simulink model "Lorien"  (R2014a)
settings: Solver=ode45  StartTime=0.0  StopTime=inf  FixedStep=0.05  RelTol=1e-3
undefined symbols (not defined in the file or in its folder): dotSelection
settings Model: Creator=Ilya  LastModifiedBy=Ilya
settings OptimizationCC: InitFltsAndDblsToZero=on
settings DebuggingCC: SaveWithParameterizedLinksMsg=none  UnderspecifiedInitializationDetection=Classic  SignalResolutionControl=TryResolveAllWithWarning  MultiTaskDSMMsg=warning  MultiTaskCondExecSysMsg=none
settings SFSimCC: SimParseCustomCode=off
settings RTWCC: IncludeERTFirstTime=on
settings GRTTargetCC: TargetFcnLib=ansi_tfl_tmw.mat  CombineOutputUpdateFcns=off  GRTInterface=on

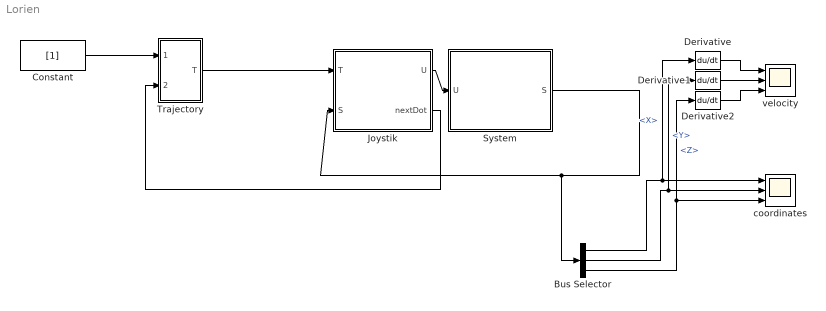
== system Lorien ==
  Bus Selector : BusSelector  DialogController=Simulink.DDGSource_Bus  OutputSignals=X,Y,Z
  Constant : Constant  Value=[1]
  Derivative : Derivative
  Derivative1 : Derivative
  Derivative2 : Derivative
  "Joystik " : Subsystem
  System : Subsystem  mask{X0=[10, 25, 2], WorkArea=[50, 20, 15], Platform=[2, 1.2]}
      mask prompts: X0 "Initial position [x, y, z] (m)"; WorkArea "Work area size [a, b, h] (m)"; Platform "Platform size [d, f]"
      mask init:
      | a = WorkArea(1);
      | b = WorkArea(2);
      | h = WorkArea(3);
      | 
      | d = Platform(1);
      | f = Platform(2);
      | 
      | L0 = iSolver(X0, a, b, d, f, h);
  Trajectory : Subsystem  mask{i=1}
      mask prompts: i "Iteration [i]"
  coordinates : Scope  NumInputPorts=3
      settings: TimeRange=10  YMin=9.5~23.75~0.967081  YMax=10.5~26.25~1.06888  SaveName=ScopeData2
  velocity : Scope  NumInputPorts=3
      settings: TimeRange=10  YMin=9.75~-5~4.975  YMax=11.75~5~5.2
  wires:
  "Joystik "/1(U) -> System/1(U)
  System/1(S) -> "Joystik "/2(S), Bus Selector/1
  Bus Selector/1 -> Derivative/1, coordinates/1  "<X>"
  Bus Selector/2 -> Derivative1/1, coordinates/2  "<Y>"
  Bus Selector/3 -> coordinates/3, Derivative2/1  "<Z>"
  Derivative/1 -> velocity/1
  Derivative1/1 -> velocity/2
  Derivative2/1 -> velocity/3
  Constant/1 -> Trajectory/1(trSelect)
  "Joystik "/2(nextDot) -> Trajectory/2(nextDot)
  Trajectory/1(T) -> "Joystik "/1(T)

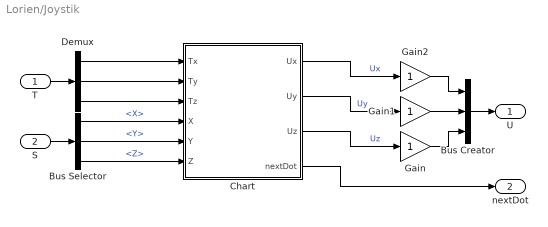
== system Lorien/Joystik  ==
  T : Inport
  S : Inport  Port=2
  Bus Creator : BusCreator  DialogController=Simulink.DDGSource_Bus  Inputs=3
  Bus Selector : BusSelector  DialogController=Simulink.DDGSource_Bus  OutputSignals=X,Y,Z
  Chart : Stateflow chart  TreatAsAtomicUnit=on
  Demux : Demux  Outputs=3
  Gain : Gain
  Gain1 : Gain
  Gain2 : Gain
  U : Outport
  nextDot : Outport  Port=2
  wires:
  Bus Creator/1 -> U/1
  S/1 -> Bus Selector/1
  Bus Selector/1 -> Chart/4(X)  "<X>"
  Bus Selector/2 -> Chart/5(Y)  "<Y>"
  Bus Selector/3 -> Chart/6(Z)  "<Z>"
  Chart/1(Ux) -> Gain2/1  "Ux"
  Chart/2(Uy) -> Gain1/1  "Uy"
  Chart/3(Uz) -> Gain/1  "Uz"
  T/1 -> Demux/1
  Demux/1 -> Chart/1(Tx)
  Demux/2 -> Chart/2(Ty)
  Demux/3 -> Chart/3(Tz)
  Gain/1 -> Bus Creator/3
  Gain1/1 -> Bus Creator/2
  Gain2/1 -> Bus Creator/1
  Chart/4(nextDot) -> nextDot/1

== system Lorien/System ==
  U : Inport
  Controller : Subsystem
  Kranes : Subsystem
      mask init:
      | T=0.1;
  Monitor : Subsystem  mask{B=on, X0=X0, A=WorkArea, P=Platform, S=15, U=1}
      mask prompts: B "Enable animation"; X0 "Initial position [x,y,z] (m)"; A "Area size [a, b, h] (m)"; P "Platform size [f, d] (m)"; S "Scale"; U "Update time (sec)"
      mask init:
      | Config.a = A(1);
      | Config.b = A(2);
      | Config.h = A(3);
      | Config.f = P(1);
      | Config.d = P(2);
      | Config.E = B;
      | Config.S = S;
      | Config.U = U;
      | Config.X0 = X0;
  S : Outport
  wires:
  Controller/1(Q) -> Kranes/1(Q)
  Kranes/1(L) -> Controller/1(L)
  Controller/2(S) -> S/1, Monitor/1(S)
  U/1 -> Controller/2(U)

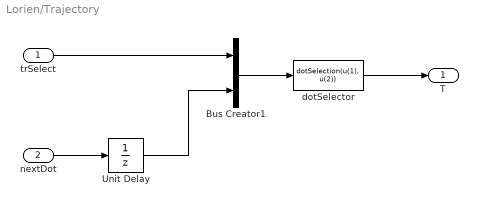
== system Lorien/Trajectory ==
  trSelect : Inport
  nextDot : Inport  Port=2
  Bus Creator1 : BusCreator  Inputs=2
  Unit Delay : UnitDelay  SampleTime=-1
  dotSelector : MATLABFcn  MATLABFcn=dotSelection(u(1), u(2))  OutputDimensions=3
  T : Outport
  wires:
  nextDot/1 -> Unit Delay/1
  Unit Delay/1 -> Bus Creator1/2
  trSelect/1 -> Bus Creator1/1
  dotSelector/1 -> T/1
  Bus Creator1/1 -> dotSelector/1

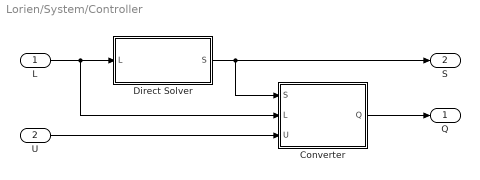
== system Lorien/System/Controller ==
  L : Inport
  U : Inport  Port=2
  Converter : Subsystem
  Direct Solver : Subsystem
  Q : Outport
  S : Outport  Port=2
  wires:
  U/1 -> Converter/3(U)
  Converter/1(Q) -> Q/1
  L/1 -> Direct Solver/1(L), Converter/2(L)
  Direct Solver/1(S) -> S/1, Converter/1(S)

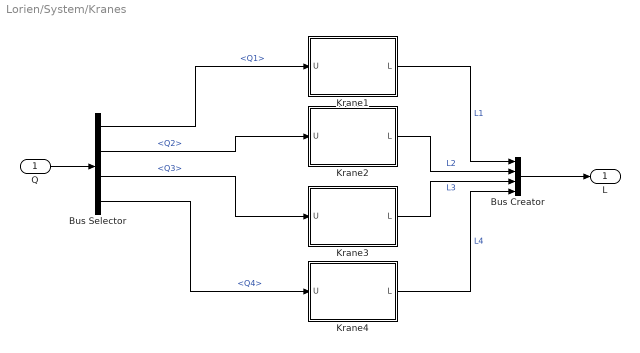
== system Lorien/System/Kranes ==
  Q : Inport
  Bus Creator : BusCreator  DialogController=Simulink.DDGSource_Bus
  Bus Selector : BusSelector  DialogController=Simulink.DDGSource_Bus  OutputSignals=Q1,Q2,Q3,Q4
  Krane1 : Subsystem  mask{IC=L0(1), T=T, D=0.5}
      mask prompts: IC "Initial condition"; D "Winch diameter (m)"
  Krane2 : Subsystem  mask{IC=L0(1), T=T, D=0.5}
      mask prompts: IC "Initial condition"; D "Winch diameter (m)"
  Krane3 : Subsystem  mask{IC=L0(1), T=T, D=0.5}
      mask prompts: IC "Initial condition"; D "Winch diameter (m)"
  Krane4 : Subsystem  mask{IC=L0(1), T=T, D=0.5}
      mask prompts: IC "Initial condition"; D "Winch diameter (m)"
  L : Outport
  wires:
  Bus Creator/1 -> L/1
  Krane1/1(L) -> Bus Creator/1  "L1"
  Krane2/1(L) -> Bus Creator/2  "L2"
  Krane3/1(L) -> Bus Creator/3  "L3"
  Krane4/1(L) -> Bus Creator/4  "L4"
  Q/1 -> Bus Selector/1
  Bus Selector/1 -> Krane1/1(U)  "<Q1>"
  Bus Selector/2 -> Krane2/1(U)  "<Q2>"
  Bus Selector/3 -> Krane3/1(U)  "<Q3>"
  Bus Selector/4 -> Krane4/1(U)  "<Q4>"

== system Lorien/System/Monitor ==
  S : Inport
  S-Function : S-Function  FunctionName=Animation  Parameters=Config  EnableBusSupport=off
  wires:
  S/1 -> S-Function/1

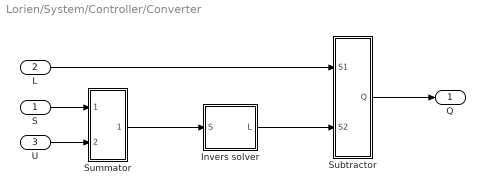
== system Lorien/System/Controller/Converter ==
  S : Inport
  L : Inport  Port=2
  U : Inport  Port=3
  Invers solver : Subsystem
  Subtractor : Subsystem
      mask Display: disp('sub')
  Summator : Subsystem
      mask Display: disp('sum')
  Q : Outport
  wires:
  Summator/1(SUM) -> Invers solver/1(S)
  Invers solver/1(L) -> Subtractor/2(S2)
  S/1 -> Summator/1(S1)
  L/1 -> Subtractor/1(S1)
  Subtractor/1(Q) -> Q/1
  U/1 -> Summator/2(S2)

== system Lorien/System/Controller/Direct Solver ==
  L : Inport
  Bus Creator : BusCreator  DialogController=Simulink.DDGSource_Bus  Inputs=3
  Demux : Demux  Outputs=3
  MATLAB Fcn : MATLABFcn  MATLABFcn=dSolver(u, a, b, d, f, h)  OutputDimensions=3
  S : Outport
  wires:
  L/1 -> MATLAB Fcn/1
  MATLAB Fcn/1 -> Demux/1
  Demux/1 -> Bus Creator/1  "X"
  Demux/2 -> Bus Creator/2  "Y"
  Demux/3 -> Bus Creator/3  "Z"
  Bus Creator/1 -> S/1

== system Lorien/System/Kranes/Krane1 ==
  U : Inport
  Motor : Subsystem
      mask Display: plot(-80,-80,80,80,[0,9,18,24,29,30,29,24,18,9,0,-9,-18,-24,-29,-30,-29,-24,-18,-9,0],[30,29,24,18,9,0,-9,-18,-24,-29,-30,-29,-24,-18,-9,0,9,18,24,29,30],[-29,-35,-35,-29],[-8,-8,8,8],[29,35,35,29],[-8,-8,8,8],[-35,-55],[0,0],[35,55],[0,0],[-78,-50,-50,-49,-45,-39,-33,-26,-21,-18,-17,-19,-22,-22,-26,-27,-25,-22,-16,-9,-3,2,6,6,4,1,1,-3,-4,-2,2,7,14,20,26,29,30,28,24,24,21,20,21,25,31,37,44,49,50,50,50,78]*.7,[58,58,57.2,49.2,42.8,38.8,38,39.6,44.4,51.6,59.6,67.6,72.4,72.4,65.2,57.2,49.2,42.8,38.8,38,39.6,44.4,51.6,59.6,67.6,72.4,72.4,65.2,57.2,49.2,42.8,38.8,38,39.6,44.4,51.6,59.6,67.6,72.4,72.4,65.2,57.2,49.2,42.8,38.8,38,39.6,44.4,51.6,58,58,58]*.6+15 );
  Winch : Subsystem
  L : Outport
  wires:
  Motor/1(Alpha) -> Winch/1(Alpha)
  Winch/1(L) -> L/1
  U/1 -> Motor/1(U)

== system Lorien/System/Kranes/Krane2 ==
  U : Inport
  Motor : Subsystem
      mask Display: plot(-80,-80,80,80,[0,9,18,24,29,30,29,24,18,9,0,-9,-18,-24,-29,-30,-29,-24,-18,-9,0],[30,29,24,18,9,0,-9,-18,-24,-29,-30,-29,-24,-18,-9,0,9,18,24,29,30],[-29,-35,-35,-29],[-8,-8,8,8],[29,35,35,29],[-8,-8,8,8],[-35,-55],[0,0],[35,55],[0,0],[-78,-50,-50,-49,-45,-39,-33,-26,-21,-18,-17,-19,-22,-22,-26,-27,-25,-22,-16,-9,-3,2,6,6,4,1,1,-3,-4,-2,2,7,14,20,26,29,30,28,24,24,21,20,21,25,31,37,44,49,50,50,50,78]*.7,[58,58,57.2,49.2,42.8,38.8,38,39.6,44.4,51.6,59.6,67.6,72.4,72.4,65.2,57.2,49.2,42.8,38.8,38,39.6,44.4,51.6,59.6,67.6,72.4,72.4,65.2,57.2,49.2,42.8,38.8,38,39.6,44.4,51.6,59.6,67.6,72.4,72.4,65.2,57.2,49.2,42.8,38.8,38,39.6,44.4,51.6,58,58,58]*.6+15 );
  Winch : Subsystem
  L : Outport
  wires:
  U/1 -> Motor/1(U)
  Winch/1(L) -> L/1
  Motor/1(Alpha) -> Winch/1(Alpha)

== system Lorien/System/Kranes/Krane3 ==
  U : Inport
  Motor : Subsystem
      mask Display: plot(-80,-80,80,80,[0,9,18,24,29,30,29,24,18,9,0,-9,-18,-24,-29,-30,-29,-24,-18,-9,0],[30,29,24,18,9,0,-9,-18,-24,-29,-30,-29,-24,-18,-9,0,9,18,24,29,30],[-29,-35,-35,-29],[-8,-8,8,8],[29,35,35,29],[-8,-8,8,8],[-35,-55],[0,0],[35,55],[0,0],[-78,-50,-50,-49,-45,-39,-33,-26,-21,-18,-17,-19,-22,-22,-26,-27,-25,-22,-16,-9,-3,2,6,6,4,1,1,-3,-4,-2,2,7,14,20,26,29,30,28,24,24,21,20,21,25,31,37,44,49,50,50,50,78]*.7,[58,58,57.2,49.2,42.8,38.8,38,39.6,44.4,51.6,59.6,67.6,72.4,72.4,65.2,57.2,49.2,42.8,38.8,38,39.6,44.4,51.6,59.6,67.6,72.4,72.4,65.2,57.2,49.2,42.8,38.8,38,39.6,44.4,51.6,59.6,67.6,72.4,72.4,65.2,57.2,49.2,42.8,38.8,38,39.6,44.4,51.6,58,58,58]*.6+15 );
  Winch : Subsystem
  L : Outport
  wires:
  Motor/1(Alpha) -> Winch/1(Alpha)
  Winch/1(L) -> L/1
  U/1 -> Motor/1(U)

== system Lorien/System/Kranes/Krane4 ==
  U : Inport
  Motor : Subsystem
      mask Display: plot(-80,-80,80,80,[0,9,18,24,29,30,29,24,18,9,0,-9,-18,-24,-29,-30,-29,-24,-18,-9,0],[30,29,24,18,9,0,-9,-18,-24,-29,-30,-29,-24,-18,-9,0,9,18,24,29,30],[-29,-35,-35,-29],[-8,-8,8,8],[29,35,35,29],[-8,-8,8,8],[-35,-55],[0,0],[35,55],[0,0],[-78,-50,-50,-49,-45,-39,-33,-26,-21,-18,-17,-19,-22,-22,-26,-27,-25,-22,-16,-9,-3,2,6,6,4,1,1,-3,-4,-2,2,7,14,20,26,29,30,28,24,24,21,20,21,25,31,37,44,49,50,50,50,78]*.7,[58,58,57.2,49.2,42.8,38.8,38,39.6,44.4,51.6,59.6,67.6,72.4,72.4,65.2,57.2,49.2,42.8,38.8,38,39.6,44.4,51.6,59.6,67.6,72.4,72.4,65.2,57.2,49.2,42.8,38.8,38,39.6,44.4,51.6,59.6,67.6,72.4,72.4,65.2,57.2,49.2,42.8,38.8,38,39.6,44.4,51.6,58,58,58]*.6+15 );
  Winch : Subsystem
  L : Outport
  wires:
  U/1 -> Motor/1(U)
  Winch/1(L) -> L/1
  Motor/1(Alpha) -> Winch/1(Alpha)

== system Lorien/System/Controller/Converter/Invers solver ==
  S : Inport
  Bus Creator : BusCreator  DialogController=Simulink.DDGSource_Bus
  Demux : Demux
  MATLAB Fcn : MATLABFcn  MATLABFcn=iSolver(u, a, b, d, f, h)  OutputDimensions=4
  L : Outport
  wires:
  Demux/1 -> Bus Creator/1  "L1"
  Demux/2 -> Bus Creator/2  "L2"
  Demux/3 -> Bus Creator/3  "L3"
  Demux/4 -> Bus Creator/4  "L4"
  Bus Creator/1 -> L/1
  S/1 -> MATLAB Fcn/1
  MATLAB Fcn/1 -> Demux/1

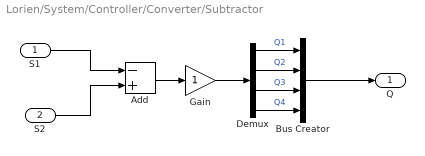
== system Lorien/System/Controller/Converter/Subtractor ==
  S1 : Inport
  S2 : Inport  Port=2
  Add : Sum  Inputs=-+
  Bus Creator : BusCreator  DialogController=Simulink.DDGSource_Bus
  Demux : Demux
  Gain : Gain
  Q : Outport
  wires:
  Demux/3 -> Bus Creator/3  "Q3"
  Demux/2 -> Bus Creator/2  "Q2"
  Demux/1 -> Bus Creator/1  "Q1"
  Add/1 -> Gain/1
  S2/1 -> Add/2
  S1/1 -> Add/1
  Demux/4 -> Bus Creator/4  "Q4"
  Gain/1 -> Demux/1
  Bus Creator/1 -> Q/1

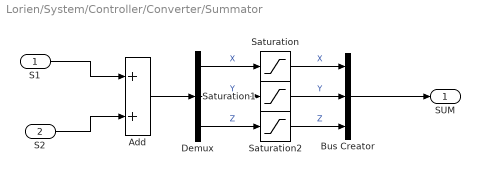
== system Lorien/System/Controller/Converter/Summator ==
  S1 : Inport
  S2 : Inport  Port=2
  Add : Sum
  Bus Creator : BusCreator  DialogController=Simulink.DDGSource_Bus  Inputs=3
  Demux : Demux  Outputs=3
  Saturation : Saturate  UpperLimit=b-f/2  LowerLimit=f/2
  Saturation1 : Saturate  UpperLimit=a-d/2  LowerLimit=d/2
  Saturation2 : Saturate  UpperLimit=h  LowerLimit=0
  SUM : Outport
  wires:
  S1/1 -> Add/1
  S2/1 -> Add/2
  Add/1 -> Demux/1
  Bus Creator/1 -> SUM/1
  Demux/1 -> Saturation/1  "X"
  Demux/2 -> Saturation1/1  "Y"
  Demux/3 -> Saturation2/1  "Z"
  Saturation/1 -> Bus Creator/1  "X"
  Saturation1/1 -> Bus Creator/2  "Y"
  Saturation2/1 -> Bus Creator/3  "Z"

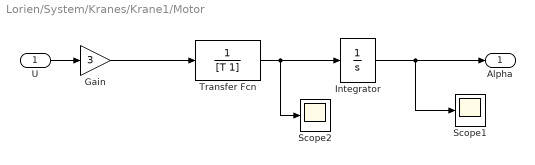
== system Lorien/System/Kranes/Krane1/Motor ==
  U : Inport
  Gain : Gain  Gain=3
  Integrator : Integrator  InitialCondition=2*IC/D
  Scope1 : Scope
      settings: YMin=111.659  YMax=111.659
  Scope2 : Scope
      settings: YMin=2.47e-010  YMax=2.555e-010  SaveName=ScopeData3
  Transfer Fcn : TransferFcn  Denominator=[T 1]
  Alpha : Outport
  wires:
  U/1 -> Gain/1
  Integrator/1 -> Alpha/1, Scope1/1
  Gain/1 -> Transfer Fcn/1
  Transfer Fcn/1 -> Integrator/1, Scope2/1

== system Lorien/System/Kranes/Krane1/Winch ==
  Alpha : Inport
  Gain : Gain  Gain=D/2
  L : Outport
  wires:
  Alpha/1 -> Gain/1
  Gain/1 -> L/1

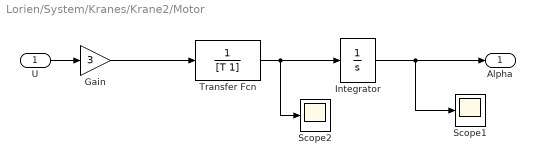
== system Lorien/System/Kranes/Krane2/Motor ==
  U : Inport
  Gain : Gain  Gain=3
  Integrator : Integrator  InitialCondition=2*IC/D
  Scope1 : Scope
  Scope2 : Scope
      settings: YMin=2.47e-010  YMax=2.555e-010  SaveName=ScopeData3
  Transfer Fcn : TransferFcn  Denominator=[T 1]
  Alpha : Outport
  wires:
  Transfer Fcn/1 -> Scope2/1, Integrator/1
  Gain/1 -> Transfer Fcn/1
  Integrator/1 -> Scope1/1, Alpha/1
  U/1 -> Gain/1

== system Lorien/System/Kranes/Krane2/Winch ==
  Alpha : Inport
  Gain : Gain  Gain=D/2
  L : Outport
  wires:
  Gain/1 -> L/1
  Alpha/1 -> Gain/1

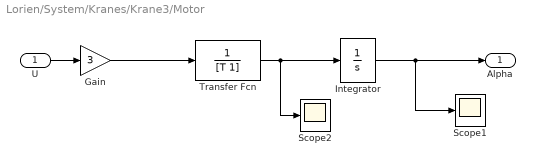
== system Lorien/System/Kranes/Krane3/Motor ==
  U : Inport
  Gain : Gain  Gain=3
  Integrator : Integrator  InitialCondition=2*IC/D
  Scope1 : Scope
  Scope2 : Scope
      settings: YMin=2.47e-010  YMax=2.555e-010  SaveName=ScopeData3
  Transfer Fcn : TransferFcn  Denominator=[T 1]
  Alpha : Outport
  wires:
  U/1 -> Gain/1
  Integrator/1 -> Alpha/1, Scope1/1
  Gain/1 -> Transfer Fcn/1
  Transfer Fcn/1 -> Integrator/1, Scope2/1

== system Lorien/System/Kranes/Krane3/Winch ==
  Alpha : Inport
  Gain : Gain  Gain=D/2
  L : Outport
  wires:
  Alpha/1 -> Gain/1
  Gain/1 -> L/1

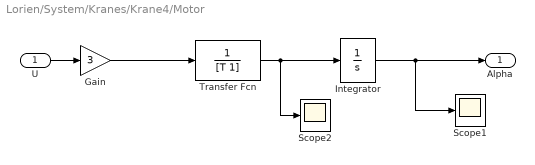
== system Lorien/System/Kranes/Krane4/Motor ==
  U : Inport
  Gain : Gain  Gain=3
  Integrator : Integrator  InitialCondition=2*IC/D
  Scope1 : Scope
  Scope2 : Scope
      settings: YMin=2.47e-010  YMax=2.555e-010  SaveName=ScopeData3
  Transfer Fcn : TransferFcn  Denominator=[T 1]
  Alpha : Outport
  wires:
  Transfer Fcn/1 -> Scope2/1, Integrator/1
  Gain/1 -> Transfer Fcn/1
  Integrator/1 -> Scope1/1, Alpha/1
  U/1 -> Gain/1

== system Lorien/System/Kranes/Krane4/Winch ==
  Alpha : Inport
  Gain : Gain  Gain=D/2
  L : Outport
  wires:
  Gain/1 -> L/1
  Alpha/1 -> Gain/1

== stateflow chart Lorien/Joystik /Chart ==
  state Idle
  (default) -> Idle
  (junction 41) -> Idle [order 1] : {Ux=0;Uy=0;Uz=0; nextDot =nextDot + 1;}
  (junction 30) -> (junction 41) [order 2]
  (junction 41) -> ? [order 1]
  (junction 34) -> Idle
  (junction 39) -> Idle : {Ux=0;Uy=0;}
  Idle -> (junction 30)
  (junction 30) -> (junction 31) [order 1] : [mod(X-Tx) > D/S | mod(Y-Ty) > D/S | (mod(Z-Tz) > D/S & S>1) ]
  (junction 40) -> (junction 39) [order 2] : [Z<0]{Uz=1;}
  (junction 31) -> ? [order 1] : [S==1]
  (junction 31) -> (junction 38) [order 1]
  (junction 40) -> (junction 39) [order 1] : [Z>6]{Uz=-1;}
  (junction 38) -> (junction 32) [order 2] : {Uz=0;}
  (junction 38) -> (junction 33) [order 1] : [mod(Z-Tz) > D/S]
  (junction 40) -> (junction 32) [order 3] : {Uz=0;}
  (junction 33) -> (junction 32) [order 2] : {Uz=1;}
  (junction 33) -> (junction 32) [order 1] : [Z>Tz]{Uz=-1;}
  (junction 32) -> (junction 35) [order 2] : {Ux=0;}
  (junction 32) -> (junction 36) [order 1] : [mod(X-Tx) > D/S]
  (junction 36) -> (junction 35) [order 2] : {Ux=-1;}
  (junction 36) -> (junction 35) [order 1] : [X<Tx]{Ux=1;}
  (junction 35) -> (junction 34) [order 2] : {Uy=0;}
  (junction 35) -> (junction 37) [order 1] : [mod(Y-Ty) > D/S]
  (junction 37) -> (junction 34) [order 2] : {Uy=-1;}
  (junction 37) -> (junction 34) [order 1] : [Y<Ty]{Uy=1;}
  data: X function_input double; Y function_output double; Ux output double; Uy output double; Uz output double; Tx input double; Ty input double; Tz input double; X input double; Y input double; Z input double; D constant double =0.1; S local double =1; nextDot output double =1
  function Y = mod(X):
    | function Y = mod(X)
    |     
    |   Y = abs(X);
